simulink model "adc_only"  (R2021a)
settings: Solver=VariableStepAuto  StartTime=0.0  StopTime=10.0  RelTol=1e-3
undefined symbols (not defined in the file): datetime, posixtime
libraries: xbsIndex_r4 x450, casper_library_misc x2, xps_library x1
(part 1 of 7)
settings Model: Creator=jackh  LastModifiedBy=jackh

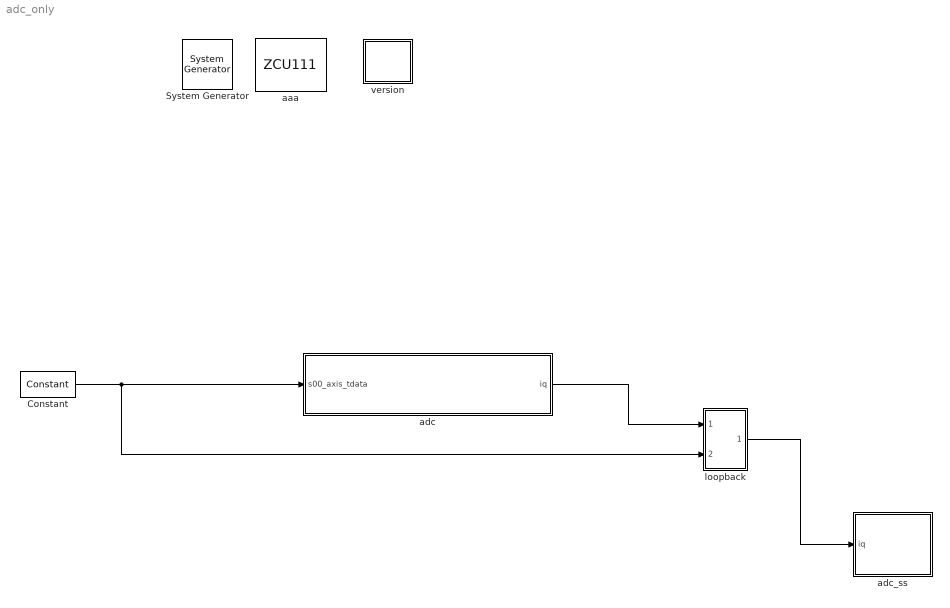
== system adc_only ==
  " System Generator" : xbsIndex_r4/ System Generator  Tag=genX  xilinxfamily=zynquplusRFSOC  part=xczu28dr  speed=-2-e  package=ffvg1517  synthesis_tool=XST  clock_wrapper=Clock Enables  directory=/home/jackh/src/souk-firmware/firmware/adc_only/sysgen  proj_type=Vivado  Synth_file=Vivado Synthesis Defaults  Impl_file=Vivado Implementation Defaults  testbench=off  simulink_period=1  sysclk_period=3.2  dcm_input_clock_period=10  incr_netlist=off  trim_vbits=Everywhere in SubSystem  dbl_ovrd=According to Block Masks  core_generation=According to Block Masks  run_coregen=off  deprecated_control=off  eval_field=0  block_type=sysgen
  Constant : xbsIndex_r4/Constant  const=0  gui_display_data_type=Fixed-point  arith_type=Unsigned  n_bits=16*8*2  bin_pt=0  preci_type=Single  exp_width=8  frac_width=24  explicit_period=on  period=1  equ=P=C  opselect=C  inp2=PCIN>>17  opr=+  inp1=P  carry=CIN  dbl_ovrd=off  block_type=constant
  aaa : xps_library/Platforms/ZCU111  Tag=xps:xsg  hw_sys=ZCU111:xczu28dr  clk_src=adc_clk  clk_rate=312.5  pl_clk_rate=125  sample_period=1  synthesis_tool=XST
      settings: SourceProductName=CASPER XPS Blockset
  adc : Subsystem
  adc_ss : Subsystem
  loopback : Subsystem
  version : Subsystem  mask{fw_type=0, ver_maj=1, ver_min=0, ver_rev=0, ver_bugfix=0}
      mask prompts: fw_type "Firmware Type"; ver_maj "Major version"; ver_min "Minor version"; ver_rev "Revision"; ver_bugfix "Bugfix"
  wires:
  Constant/1 -> loopback/2(dac), adc/1(s00_axis_tdata)
  loopback/1(out) -> adc_ss/1(iq)
  adc/1(iq) -> loopback/1(adc)
